simulink model "Assignment_1"  (R2022b)
settings: Solver=FixedStepAuto  StartTime=0.0  StopTime=100  FixedStep=1e-3  RelTol=1e-3  EnableMultiTasking=on
undefined symbols (not defined in the file): D1, D10, D11, D12, D13, D2, D3, D5, D8, D9, PTA0, PTA1, PTA2, PTB9, PTC17, PTC4, PTD0, PTD1, PTD2, PTD3
libraries: frdmk64flib x10
settings Model: ExtModeTrigDuration=5  Creator=aldenluscher  LastModifiedBy=aldenluscher
settings OptimizationCC: EnhancedBackFolding=on  PassReuseOutputArgsAs=Individual arguments  ZeroExternalMemoryAtStartup=off  ZeroInternalMemoryAtStartup=off  MaxStackSize=64  OptimizeBlockOrder=speed  DifferentSizesBufferReuse=on  OptimizationCustomize=off  EfficientTunableParamExpr=on
settings DebuggingCC: ParameterTunabilityLossMsg=error
settings HardwareCC: ProdBitPerPointer=32  ProdBitPerSizeT=32  ProdBitPerPtrDiffT=32  ProdLargestAtomicInteger=Long  ProdLargestAtomicFloat=Double  ProdWordSize=32  ProdHWDeviceType=ARM Compatible->ARM Cortex
settings SFSimCC: MATLABDynamicMemAlloc=off
settings RTWCC: Description=Embedded Coder  SystemTargetFile=ert.tlc  HardwareBoard=NXP FRDM-K64F  TLCOptions="-aInlineSetEventsForThisBaseRateFcn=TLC_FALSE -aSuppressMultiTaskScheduler=TLC_FALSE  -aRateBasedStepFcn=0"  TemplateMakefile=ert_default_tmf  Toolchain=GNU Tools for ARM Embedded Processors
settings CodeAppCC: ForceParamTrailComments=on  IgnoreCustomStorageClasses=off  OperatorAnnotations=on  SimulinkDataObjDesc=on  SFDataObjDesc=on  InsertBlockDesc=on
settings ERTTargetCC: ExtModeTransport=4  ExtModeMexFile=sendToCommService

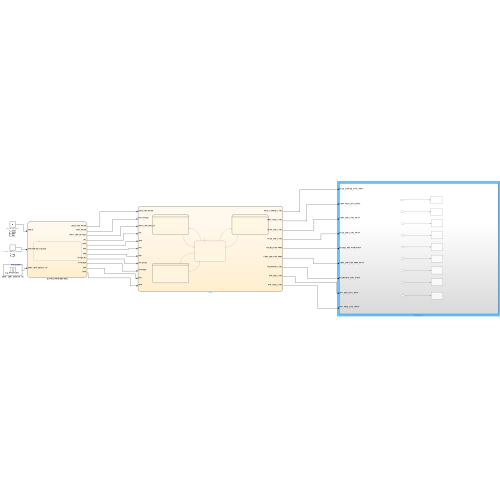
[thumbnail: Simulink's stored preview of the top-level diagram]
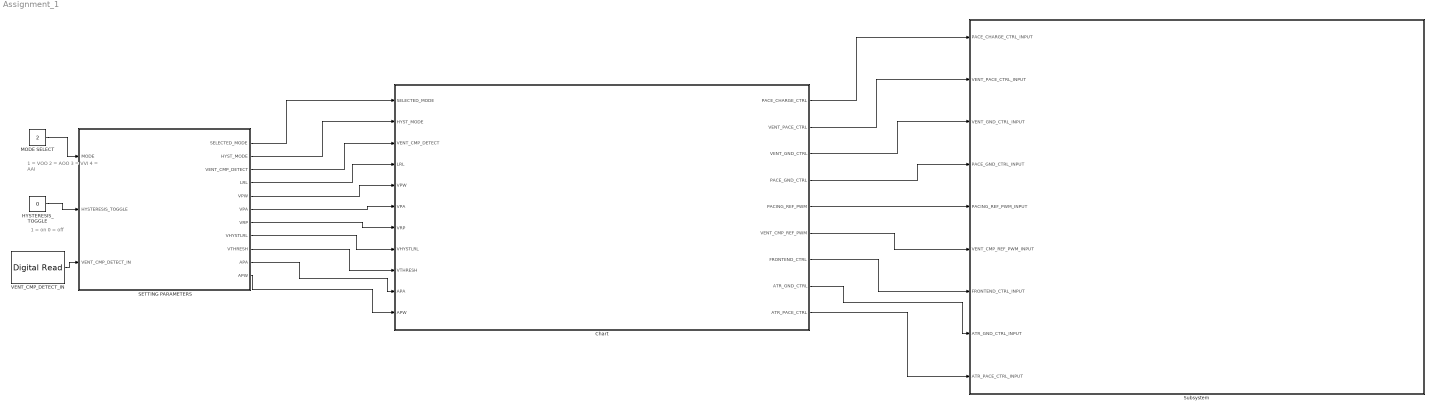
== system Assignment_1 ==
  note: 1 = VOO
      | 2 = AOO
      | 3 = VVI
      | 4 = AAI
  note: 1 = on
      | 0 = off
  Chart : Stateflow chart  TreatAsAtomicUnit=on
      settings: PortSchema="{\"entries\":[{\"content\":{\"sides\":[{\"content\":{\"connectorIds\":[\"In7\",\"In9\",\"In6\",\"In8\",\"In3\",\"In4\",\"In2\",\"In5\",\"In1\",\"In10\",\"In11\"]},\"type\":\"ConnectorPlacement.EquallySpacedRectSide\",\"uuid\":\"804be3be-5f9e-4b62-b5c8-dc084235daae\"},{\"content\":{\"connectorIds\":[\"Out1\",\"Out2\",\"Out3\",\"Out4\",\"Out5\",\"Out6\",\"Out7\",\"Out8\",\"Out9\"],\"side\":\"RIGHT\"},\"type\":\"ConnectorPlacement.EquallySpacedRectSide\",\"uuid\":\"906acfdb-1dc8-44fd-8d51-f28f98719a27\"},{\"content\":{\"connectorIds\":[],\"side\":\"TOP\"},\"type\":\"ConnectorPlacement.EquallySpacedRectSide\",\"uuid\":\"8d057b55-2cbd-487f-8484-177f9fa59c90\"}]},\"type\":\"ConnectorPlacement.EquallySpacedConnector\",\"uuid\":\"d5bd6f86-9a36-412f-a1f0-e96663509123\"}],\"packageUris\":[\"http://schema.mathworks.com/mf0/Connector/R2020b\"],\"version\":\"1.0\"}"
  HYSTERESIS_TOGGLE : Constant  Value=0
  MODE SELECT : Constant  Value=2
  SETTING PARAMETERS : Stateflow chart  TreatAsAtomicUnit=on
      settings: PortSchema="{\"entries\":[{\"content\":{\"sides\":[{\"content\":{\"connectorIds\":[\"In1\",\"In2\",\"In3\"]},\"type\":\"ConnectorPlacement.EquallySpacedRectSide\",\"uuid\":\"3aca0bd7-629a-4c5c-b565-6ed0578fed9d\"},{\"content\":{\"connectorIds\":[\"Out7\",\"Out9\",\"Out6\",\"Out8\",\"Out3\",\"Out4\",\"Out2\",\"Out5\",\"Out1\",\"Out10\",\"Out11\"],\"side\":\"RIGHT\"},\"type\":\"ConnectorPlacement.EquallySpacedRectSide\",\"uuid\":\"ab26bc13-3a59-4dfe-8b46-0847370ad477\"},{\"content\":{\"connectorIds\":[],\"side\":\"TOP\"},\"type\":\"ConnectorPlacement.EquallySpacedRectSide\",\"uuid\":\"fc5ed4b5-9a01-4cf9-a838-586958f03313\"}]},\"type\":\"ConnectorPlacement.EquallySpacedConnector\",\"uuid\":\"c620314d-9c7d-46a3-b2b8-c6bca5c5944e\"}],\"packageUris\":[\"http://schema.mathworks.com/mf0/Connector/R2020b\"],\"version\":\"1.0\"}"
  Subsystem : Subsystem
  VENT_CMP_DETECT_IN : frdmk64flib/Digital Read  Whichpin=PTC17 (D1)  SampleTime=-1
  wires:
  MODE SELECT/1 -> SETTING PARAMETERS/1(MODE)
  HYSTERESIS_TOGGLE/1 -> SETTING PARAMETERS/2(HYSTERESIS_TOGGLE)
  VENT_CMP_DETECT_IN/1 -> SETTING PARAMETERS/3(VENT_CMP_DETECT_IN)
  Chart/4(PACE_GND_CTRL) -> Subsystem/4(PACE_GND_CTRL_INPUT)
  Chart/7(FRONTEND_CTRL) -> Subsystem/7(FRONTEND_CTRL_INPUT)
  Chart/5(PACING_REF_PWM) -> Subsystem/5(PACING_REF_PWM_INPUT)
  Chart/1(PACE_CHARGE_CTRL) -> Subsystem/1(PACE_CHARGE_CTRL_INPUT)
  Chart/3(VENT_GND_CTRL) -> Subsystem/3(VENT_GND_CTRL_INPUT)
  Chart/6(VENT_CMP_REF_PWM) -> Subsystem/6(VENT_CMP_REF_PWM_INPUT)
  Chart/2(VENT_PACE_CTRL) -> Subsystem/2(VENT_PACE_CTRL_INPUT)
  SETTING PARAMETERS/1(VTHRESH) -> Chart/1(VTHRESH)
  SETTING PARAMETERS/2(VRP) -> Chart/2(VRP)
  SETTING PARAMETERS/3(VPW) -> Chart/3(VPW)
  SETTING PARAMETERS/4(VPA) -> Chart/4(VPA)
  SETTING PARAMETERS/5(VHYSTLRL) -> Chart/5(VHYSTLRL)
  SETTING PARAMETERS/6(VENT_CMP_DETECT) -> Chart/6(VENT_CMP_DETECT)
  SETTING PARAMETERS/7(SELECTED_MODE) -> Chart/7(SELECTED_MODE)
  SETTING PARAMETERS/8(LRL) -> Chart/8(LRL)
  SETTING PARAMETERS/9(HYST_MODE) -> Chart/9(HYST_MODE)
  SETTING PARAMETERS/10(APA) -> Chart/10(APA)
  SETTING PARAMETERS/11(APW) -> Chart/11(APW)
  Chart/8(ATR_GND_CTRL) -> Subsystem/8(ATR_GND_CTRL_INPUT)
  Chart/9(ATR_PACE_CTRL) -> Subsystem/9(ATR_PACE_CTRL_INPUT)

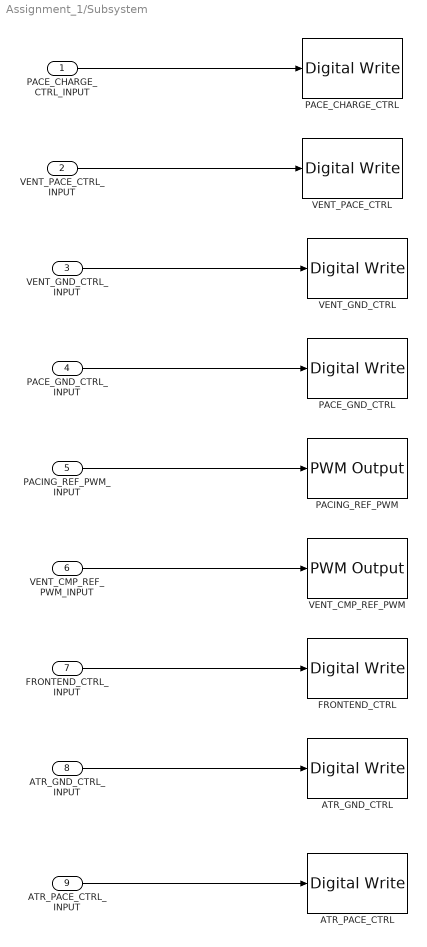
== system Assignment_1/Subsystem ==
  PACE_CHARGE_CTRL_INPUT : Inport
  VENT_PACE_CTRL_INPUT : Inport  Port=2
  VENT_GND_CTRL_INPUT : Inport  Port=3
  PACE_GND_CTRL_INPUT : Inport  Port=4
  PACING_REF_PWM_INPUT : Inport  Port=5
  VENT_CMP_REF_PWM_INPUT : Inport  Port=6
  FRONTEND_CTRL_INPUT : Inport  Port=7
  ATR_GND_CTRL_INPUT : Inport  Port=8
  ATR_PACE_CTRL_INPUT : Inport  Port=9
  ATR_GND_CTRL : frdmk64flib/Digital Write  Whichpin=PTD2 (D11)
  ATR_PACE_CTRL : frdmk64flib/Digital Write  Whichpin=PTA0 (D8)
  FRONTEND_CTRL : frdmk64flib/Digital Write  Whichpin=PTD1 (D13)
  PACE_CHARGE_CTRL : frdmk64flib/Digital Write  Whichpin=PTB9 (D2)
  PACE_GND_CTRL : frdmk64flib/Digital Write  Whichpin=PTD0 (D10)
  PACING_REF_PWM : frdmk64flib/PWM Output  Whichpin=PTA2 (D5)  InitialFrequency=2000  InitialDutyCycle=0
  VENT_CMP_REF_PWM : frdmk64flib/PWM Output  Whichpin=PTA1 (D3)  InitialFrequency=2000  InitialDutyCycle=0
  VENT_GND_CTRL : frdmk64flib/Digital Write  Whichpin=PTD3 (D12)
  VENT_PACE_CTRL : frdmk64flib/Digital Write  Whichpin=PTC4 (D9)
  wires:
  VENT_PACE_CTRL_INPUT/1 -> VENT_PACE_CTRL/1
  PACE_GND_CTRL_INPUT/1 -> PACE_GND_CTRL/1
  PACE_CHARGE_CTRL_INPUT/1 -> PACE_CHARGE_CTRL/1
  PACING_REF_PWM_INPUT/1 -> PACING_REF_PWM/1
  VENT_GND_CTRL_INPUT/1 -> VENT_GND_CTRL/1
  VENT_CMP_REF_PWM_INPUT/1 -> VENT_CMP_REF_PWM/1
  FRONTEND_CTRL_INPUT/1 -> FRONTEND_CTRL/1
  ATR_GND_CTRL_INPUT/1 -> ATR_GND_CTRL/1
  ATR_PACE_CTRL_INPUT/1 -> ATR_PACE_CTRL/1

== stateflow chart Assignment_1/SETTING PARAMETERS ==
  state Parameters_
    SELECTED_MODE = MODE; % Pacing Mode
    HYST_MODE = HYSTERESIS_TOGGLE; % Toggles On/Off Hysteresis (1 = on, 0 = off)
    VENT_CMP_DETECT = VENT_CMP_DETECT_IN; % Input value read from D1 pin
    LRL = 120; %  Lower Rate Limit (e.g. 120ppm)
    VPW = 1; % Ventricle Pulse Width
    VPA = 3.5; % Ventricle Pulse Amplitude (as voltage from 1-5V)
    VRP = 300; % Ventricle Refractory Period (msec)
    VHYSTLRL = 50; % Ventricle Hysteresis Lower Rate Limit (e.g. 50ppm)
    VTHRESH = 70; % Ventricle Pulse Detection Threshold as PWM Value (e.g 70% of 5V)
    APW = 1; % Atrial Pulse Width
    APA = 3.5; % Atrial Pulse Amplitude (as voltage from 1-5V)
  (default) -> Parameters_
  data: PACING_PERIOD local; MODE input; HYSTERESIS_TOGGLE input; VENT_CMP_DETECT_IN input; VTHRESH output; VRP output; VPW output; VPA output; VHYSTLRL output; VENT_CMP_DETECT output; SELECTED_MODE output; LRL output; HYST_MODE output; APA output; APW output

== stateflow chart Assignment_1/Chart ==
  state VOO
    state Pacing_
      PACE_CHARGE_CTRL = 0;
      PACE_GND_CTRL = 1;
      VENT_GND_CTRL = 0;
      VENT_PACE_CTRL = 1;
    state Charging_
      PACING_REF_PWM = 100*(VPA/5); % Ventricular Pulse Amplitude
      PACING_PERIOD = (60000/LRL); % Pacing Period
      PACE_CHARGE_CTRL = 1;
      PACE_GND_CTRL = 1;
      VENT_GND_CTRL = 1;
      VENT_PACE_CTRL = 0;
      %%%ATR_PACE_CTRL = 0;
      %%%ATR_GND_CTRL = 0;
    (default) -> VOO.Charging_
    VOO.Charging_ -> VOO.Pacing_ : after(PACING_PERIOD-VPW,msec)
        | %Charging time = Pacing Period - Pulse Width
    VOO.Pacing_ -> VOO.Charging_ : after(VPW,msec)
        | %Pacing time = Ventricle Pulse Width
  state VVI
    state Timing_Natural_PW_in_msec_
      NAT_PW=NAT_PW+1;
    state Refractory_Period_
      PACE_CHARGE_CTRL = 1;
      PACE_GND_CTRL = 1;
      VENT_GND_CTRL = 1;
      VENT_PACE_CTRL = 0;
    note: ATR_PACE_CTRL = false;
        | ATR_GND_CTRL = false;
    state Charging_
      PACING_REF_PWM = 100*(VPA/5); %Pulse Amplitude
      PACING_PERIOD = (60000/LRL); %Normal Pacing Period
      HYST_PERIOD = (60000/VHYSTLRL); %Hysteresis Pacing Period
      PACE_CHARGE_CTRL = 1;
      PACE_GND_CTRL = 1;
      VENT_GND_CTRL = 1;
      VENT_PACE_CTRL = 0;
      VENT_CMP_REF_PWM = VTHRESH; % Ventricle Sensing Threshold
      FRONTEND_CTRL = 1; %Sensing On
      NAT_PW = 0; % Natural Pulse Width
      TOTAL_NAT_PW = 0; % Sum of Natural Pulse
      PACE_PW = 0; % Pacemaker Pulse Width
      ARTIFICIAL = 0; % Flag to determine if a pulse was natural or artificial,
      % only has an effect when hysteresis is enabled
    state Pacing_
      PACE_CHARGE_CTRL = 0;
      PACE_GND_CTRL = 1;
      VENT_GND_CTRL = 0;
      VENT_PACE_CTRL = 1;
    state Setting_Initial_Period_
      PERIOD = (60000/LRL);
      % Period for each
      % pulse, initally set to the
      % normal PACING_PERIOD
      % but can be re-assigned to
      % the HYST_PERIOD if
      % hysteresis is enabled and
      % triggered
      %%%ATR_PACE_CTRL = 0;
      %%%ATR_GND_CTRL = 0;
      % Set ATR_PACE and
      % GND_CTRL to disabled
      % incase they were left enabled
      % from the last state
    Timing_Natural_PW_in_msec_ -> Timing_Natural_PW_in_msec_ [order 2] : after(1,msec)
        | % time the natural pulse in msec
    Timing_Natural_PW_in_msec_ -> Refractory_Period_ [order 1] : [VENT_CMP_DETECT==0]{TOTAL_NAT_PW = TOTAL_NAT_PW + NAT_PW}
        | % when the natural pulse ends add the pulsewidth of the natural pulse to the
        | % total pulsewidth of all natural pulses that have arrived while since we last
        | % paced the pacemaker
    Refractory_Period_ -> Timing_Natural_PW_in_msec_ [order 1] : [VENT_CMP_DETECT==1]{ARTIFICIAL = 0}
        | % if a natural pulse arrives while
        | % in the refractory period, the last pulse was not
        | % from the pulsemaker, and start timing the natural pulse
    Refractory_Period_ -> (junction 80) [order 2] : after(VRP-PACE_PW-TOTAL_NAT_PW,msec)
        | % after VRP-PACE_PW-TOTAL_NAT_PW then charge
    (junction 80) -> VVI.Charging_ [order 1] : [HYST_MODE == 1 && ARTIFICIAL == 0]{PERIOD = HYST_PERIOD}
        | % if hysteresis mode is on and the last pulse was a natural
        | % pulse then the pacing period for the next pulse is the HYST_PERIOD
    (junction 80) -> VVI.Charging_ [order 3] : [HYST_MODE==0]
        | % if hysteresis mode is off
    (junction 80) -> VVI.Charging_ [order 2] : [HYST_MODE == 1 && ARTIFICIAL == 1]{PERIOD = PACING_PERIOD}
        | % if hysteresis mode is on and the last pulse was sent
        | % by the pacemaker then the next pulse is the normal PACING_PERIOD
    (junction 77) -> Refractory_Period_ [order 2] : [VENT_CMP_DETECT == 1]
        | % if an incoming pulse is detected
    VVI.Pacing_ -> Refractory_Period_ : after(VPW,msec){PACE_PW = VPW, ARTIFICIAL = 1}
        | % pace for duration of VPW
    (default) -> Setting_Initial_Period_
    VVI.Charging_ -> (junction 77)
    (junction 77) -> VVI.Pacing_ [order 1] : after(PERIOD-VPW-VRP,msec)[VENT_CMP_DETECT == 0]
        | % after PERIOD-VPW-VER if no pulse is detected then pace
    Setting_Initial_Period_ -> VVI.Charging_
  state PACING_MODE_ENTRY_POINT_
  state AOO
    state Pacing_
      PACE_CHARGE_CTRL = 0;
      PACE_GND_CTRL = 1;
      ATR_GND_CTRL = 0;
      ATR_PACE_CTRL = 1;
    state Charging_
      PACING_REF_PWM = 100*(APA/5); % Atrial Pulse Amplitude
      PACING_PERIOD = (60000/LRL); % Pacing Period
      PACE_CHARGE_CTRL = 1;
      PACE_GND_CTRL = 1;
      ATR_GND_CTRL = 1;
      ATR_PACE_CTRL = 0;
      %%%VENT_GND_CTRL = 0;
      %%%VENT_PACE_CTRL = 0;
    (default) -> AOO.Charging_
    AOO.Charging_ -> AOO.Pacing_ : after(PACING_PERIOD-APW,msec)
        | %Charging time = Pacing Period - Pulse Width
    AOO.Pacing_ -> AOO.Charging_ : after(APW,msec)
        | %Pacing time = Atrial Pulse Width
  PACING_MODE_ENTRY_POINT_ -> VOO [order 2] : [SELECTED_MODE==1]
  PACING_MODE_ENTRY_POINT_ -> VVI [order 1] : [SELECTED_MODE==3]
  VOO -> PACING_MODE_ENTRY_POINT_ : [SELECTED_MODE~=1]
  VVI -> PACING_MODE_ENTRY_POINT_ : [SELECTED_MODE~=3]
  (default) -> PACING_MODE_ENTRY_POINT_
  PACING_MODE_ENTRY_POINT_ -> AOO [order 3] : [SELECTED_MODE==2]
  AOO -> PACING_MODE_ENTRY_POINT_ : [SELECTED_MODE~=2]
  data: PACE_CHARGE_CTRL output; VENT_PACE_CTRL output; VENT_GND_CTRL output; PACE_GND_CTRL output; PACING_REF_PWM output; VENT_CMP_REF_PWM output; PACING_PERIOD local; PERIOD local; HYST_PERIOD local; FRONTEND_CTRL output; NAT_PW local; TOTAL_NAT_PW local; PACE_PW local; VTHRESH input; VRP input; VPW input; VPA input; VHYSTLRL input; VENT_CMP_DETECT input; SELECTED_MODE input; LRL input; HYST_MODE input; ARTIFICIAL local; ATR_GND_CTRL output; ATR_PACE_CTRL output; APA input; APW input
